simulink model "TestChaineAirNew"  (R2025a)
settings: Solver=ode45  StartTime=0.0  StopTime=SimuPumpStop  FixedStep=0.1  MaxStep=0.005  RelTol=1e-9  EnableMultiTasking=on
undefined symbols (not defined in the file): AirMotTest, AirPapTest, AirPressureTest, AirTimeTest, gam, Mim0, nv_remp, P0, Pamb, PcolPapTest, PRcrit, Rair, RegimeTest, SectionPapTest, Tamb, TempsPapTest, TempsTest, Vcyl
settings Model: Creator=a030141  LastModifiedBy=Hugo
settings SolverCC: AlgebraicLoopSolver=TrustRegion
settings DataIOCC: LimitDataPoints=on  SaveFormat=Array  SignalLoggingSaveFormat=ModelDataLogs  ReturnWorkspaceOutputs=off  SignalLoggingName=sigsOut
settings OptimizationCC: InitFltsAndDblsToZero=on  LifeSpan=inf
settings DebuggingCC: SaveWithParameterizedLinksMsg=none  UnderspecifiedInitializationDetection=Classic  MergeDetectMultiDrivingBlocksExec=none  SignalResolutionControl=TryResolveAllWithWarning  MultiTaskDSMMsg=warning  MultiTaskCondExecSysMsg=none  FcnCallInpInsideContextMsg=warning  UnconnectedInputMsg=warning  UnconnectedOutputMsg=warning  UnconnectedLineMsg=warning  SFUnexpectedBacktrackingDiag=warning  SFNoUnconditionalDefaultTransitionDiag=warning  SFExecutionAtInitializationDiag=none  ArithmeticOperatorsInVariantConditions=warning
settings HardwareCC: ProdBitPerPointer=32.0  ProdBitPerSizeT=32.0  ProdBitPerPtrDiffT=32.0  ProdLargestAtomicFloat=None  ProdIntDivRoundTo=Undefined  ProdEndianess=Unspecified  ProdWordSize=32.0  ProdHWDeviceType=32-bit Generic  TargetUnknown=on
settings ModelReferenceCC: PropagateSignalLabelsOutOfModel=off
settings RTWCC: GPUComputeCapability=3.5
settings CodeAppCC: StateflowObjectComments=on
settings GRTTargetCC: TargetFcnLib=ansi_tfl_tmw.mat  TargetLangStandard=C89/C90 (ANSI)  CombineOutputUpdateFcns=off  GRTInterface=on
settings ConfigComp: CovMetricSettings=dw  CovSaveCumulativeToWorkspaceVar=on  CovSaveSingleToWorkspaceVar=on

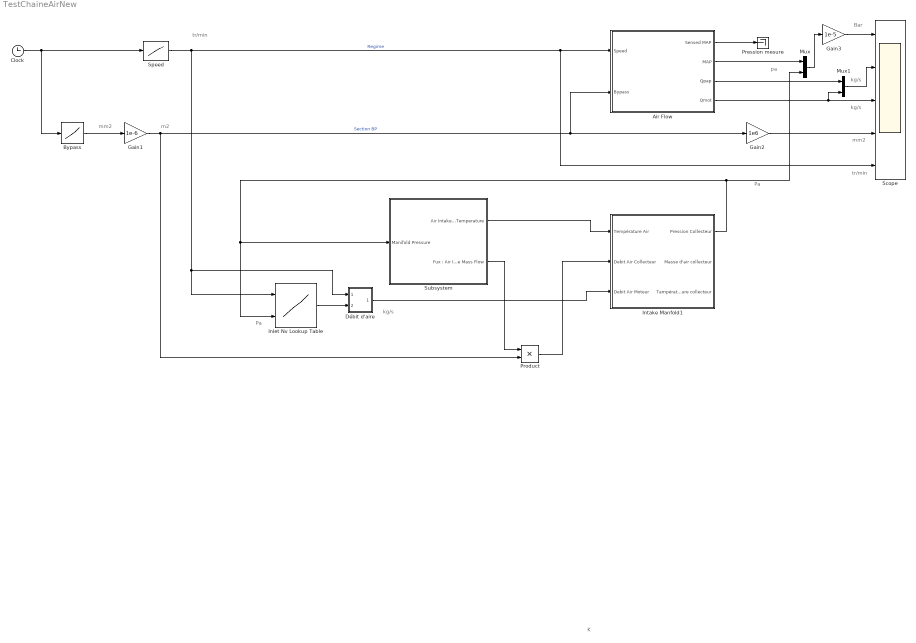
== system TestChaineAirNew ==
  note: pa
  note: Bar
  note: tr/min
  note: tr/min
  note: Pa
  note: m2
  note: mm2
  note: mm2
  note: kg/s
  note: kg/s
  note: Pa
  note: kg/s
  note: K
  Air Flow : Subsystem
  Bypass : Lookup  InputValues=TempsPapTest  Table=SectionPapTest.*PcolPapTest
  Clock : Clock
  Débit d'aire : Subsystem
  Gain1 : Gain  Gain=1e-6  SaturateOnIntegerOverflow=on  OutDataTypeStr=Inherit: Same as input  ParamDataTypeStr=Inherit: Same as input
  Gain2 : Gain  Gain=1e6  SaturateOnIntegerOverflow=on  OutDataTypeStr=Inherit: Same as input  ParamDataTypeStr=Inherit: Same as input
  Gain3 : Gain  Gain=1e-5  SaturateOnIntegerOverflow=on  OutDataTypeStr=Inherit: Same as input  ParamDataTypeStr=Inherit: Same as input
  Inlet Nv Lookup Table : Lookup2D  RowIndex=Ne_remp  ColumnIndex=Pcol_remp  Table=nv_remp
  Intake Manfold1 : Subsystem
  Mux : Mux  Inputs=2
  Mux1 : Mux  Inputs=2
  Pression mesure : Terminator
  Product : Product
  Scope : Scope  NumInputPorts=5
      settings: TimeSpan=374.5  Title=Pcol [bars]  ActiveDisplayYMinimum=0.769380841937612  ActiveDisplayYMaximum=1.0327907950597828
  Speed : Lookup  InputValues=TempsTest  Table=RegimeTest
  Subsystem : Subsystem
  wires:
  Clock/1 -> Speed/1, Bypass/1
  Bypass/1 -> Gain1/1
  Air Flow/2(MAP) -> Mux/1
  Mux/1 -> Gain3/1
  Gain3/1 -> Scope/1
  Air Flow/4(Qmot) -> Scope/3, Mux1/2
  Gain2/1 -> Scope/4
  Mux1/1 -> Scope/2
  Air Flow/1(Sensed MAP) -> Pression mesure/1
  Gain1/1 -> Gain2/1, Air Flow/2(Bypass), Product/2  "Section BP"
  Air Flow/3(Qpap) -> Mux1/1
  Speed/1 -> Scope/5, Air Flow/1(Speed), Débit d'aire/1(In1), Inlet Nv Lookup Table/1  "Regime"
  Débit d'aire/1(Debit Air Moteur) -> Intake Manfold1/3(Debit Air Moteur)
  Inlet Nv Lookup Table/1 -> Débit d'aire/2(In2)
  Subsystem/2("Fux : Air Intake Mass Flow") -> Product/1
  Product/1 -> Intake Manfold1/2(Debit Air Collecteur)
  Subsystem/1(Air Intake Temperature) -> Intake Manfold1/1(Température Air)
  Intake Manfold1/1(Pression Collecteur) -> Inlet Nv Lookup Table/2, Subsystem/1(Manifold Pressure), Mux/2

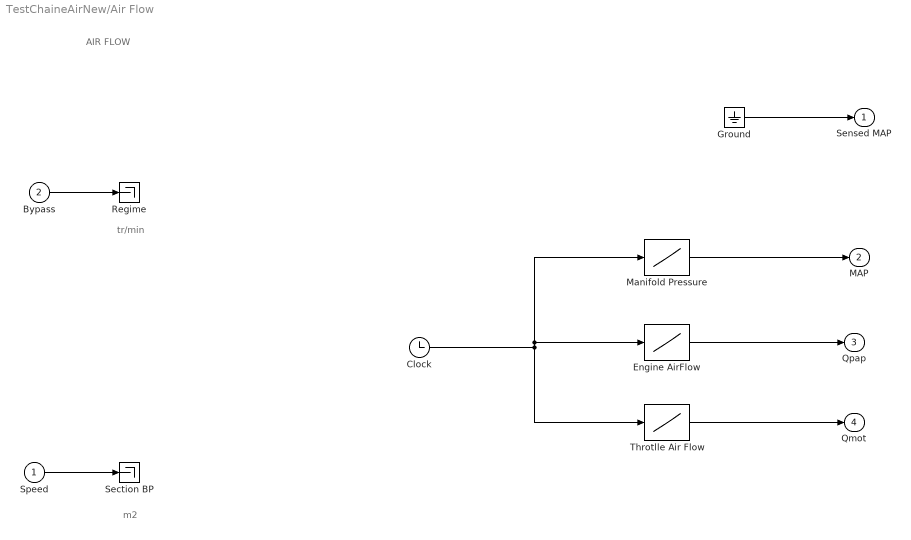
== system TestChaineAirNew/Air Flow ==
  note: AIR FLOW
  note: m2
  note: tr/min
  Speed : Inport
  Bypass : Inport  Port=2
  Clock : Clock
  Engine AirFlow : Lookup  InputValues=AirTimeTest  Table=AirMotTest
  Ground : Ground
  Manifold Pressure : Lookup  InputValues=AirTimeTest  Table=AirPressureTest
  Regime : Terminator
  Section BP : Terminator
  Throtlle Air Flow : Lookup  InputValues=AirTimeTest  Table=AirPapTest
  Sensed MAP : Outport
  MAP : Outport  Port=2
  Qpap : Outport  Port=3
  Qmot : Outport  Port=4
  wires:
  Bypass/1 -> Regime/1
  Speed/1 -> Section BP/1
  Ground/1 -> Sensed MAP/1
  Clock/1 -> Manifold Pressure/1, Engine AirFlow/1, Throtlle Air Flow/1
  Manifold Pressure/1 -> MAP/1
  Throtlle Air Flow/1 -> Qmot/1
  Engine AirFlow/1 -> Qpap/1

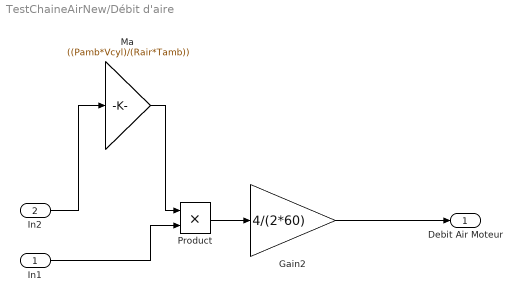
== system TestChaineAirNew/Débit d'aire ==
  In1 : Inport
  In2 : Inport  Port=2
  Gain2 : Gain  Gain=4/(2*60)
  Ma : Gain  Gain=((Pamb*Vcyl)/(Rair*Tamb))
  Product : Product
  Debit Air Moteur : Outport
  wires:
  Ma/1 -> Product/1
  Gain2/1 -> Debit Air Moteur/1
  Product/1 -> Gain2/1
  In1/1 -> Product/2
  In2/1 -> Ma/1

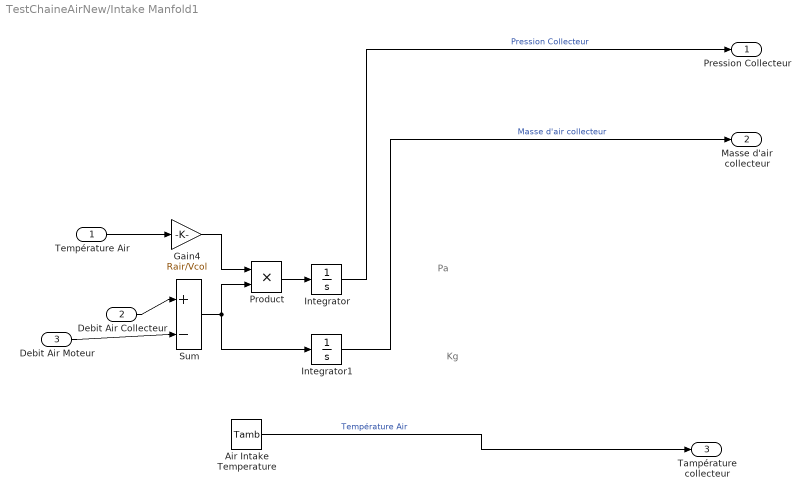
== system TestChaineAirNew/Intake Manfold1 ==
  note: Pa
  note: Kg
  Température Air : Inport
  Debit Air Collecteur : Inport  Port=2
  Debit Air Moteur : Inport  Port=3
  Air Intake Temperature : Constant  Value=Tamb
  Gain4 : Gain  Gain=Rair/Vcol
  Integrator : Integrator  InitialCondition=P0
  Integrator1 : Integrator  InitialCondition=Mim0
  Product : Product
  Sum : Sum  Inputs=|+-
  Pression Collecteur : Outport
  Masse d'air collecteur : Outport  Port=2
  Tampérature collecteur : Outport  Port=3
  wires:
  Gain4/1 -> Product/1
  Sum/1 -> Integrator1/1, Product/2
  Product/1 -> Integrator/1
  Température Air/1 -> Gain4/1
  Integrator1/1 -> Masse d'air collecteur/1  "Masse d'air collecteur"
  Debit Air Moteur/1 -> Sum/2
  Integrator/1 -> Pression Collecteur/1  "Pression Collecteur"
  Debit Air Collecteur/1 -> Sum/1
  Air Intake Temperature/1 -> Tampérature collecteur/1  "Température Air"

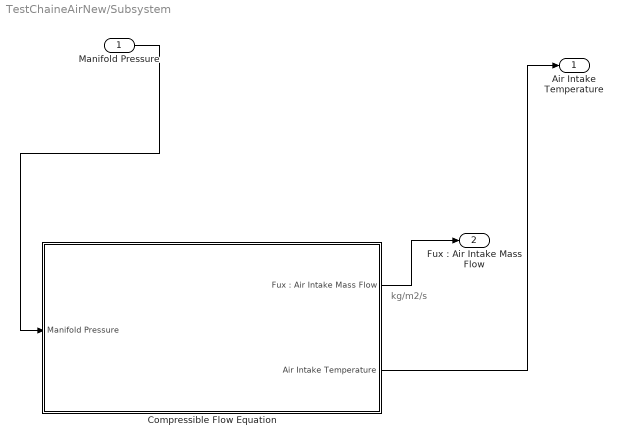
== system TestChaineAirNew/Subsystem ==
  note: kg/m2/s
  Manifold Pressure : Inport
  Compressible Flow Equation : Subsystem
  Air Intake Temperature : Outport
  "Fux : Air Intake Mass Flow" : Outport  Port=2
  wires:
  Compressible Flow Equation/2(Air Intake Temperature) -> Air Intake Temperature/1
  Manifold Pressure/1 -> Compressible Flow Equation/1(Manifold Pressure)
  Compressible Flow Equation/1("Fux : Air Intake Mass Flow") -> "Fux : Air Intake Mass Flow"/1

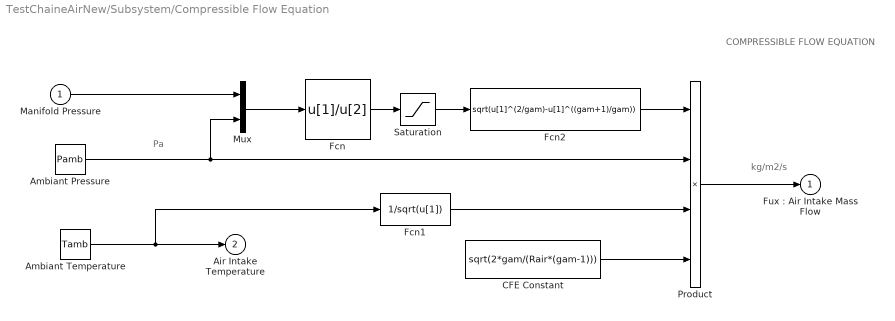
== system TestChaineAirNew/Subsystem/Compressible Flow Equation ==
  note: COMPRESSIBLE FLOW EQUATION
  note: Pa
  note: kg/m2/s
  Manifold Pressure : Inport
  Ambiant Pressure : Constant  Value=Pamb
  Ambiant Temperature : Constant  Value=Tamb
  "CFE Constant " : Constant  Value=sqrt(2*gam/(Rair*(gam-1)))
  Fcn : Fcn  Expr=u[1]/u[2]
  Fcn1 : Fcn  Expr=1/sqrt(u[1])
  Fcn2 : Fcn  Expr=sqrt(u[1]^(2/gam)-u[1]^((gam+1)/gam))
  Mux : Mux  Inputs=2
  Product : Product  Inputs=4  InputSameDT=on  SaturateOnIntegerOverflow=on  OutDataTypeStr=Inherit: Same as first input
  Saturation : Saturate  UpperLimit=1  LowerLimit=PRcrit
  "Fux : Air Intake Mass Flow" : Outport
  Air Intake Temperature : Outport  Port=2
  wires:
  Ambiant Pressure/1 -> Product/2, Mux/2
  Product/1 -> "Fux : Air Intake Mass Flow"/1
  "CFE Constant "/1 -> Product/4
  Fcn2/1 -> Product/1
  Saturation/1 -> Fcn2/1
  Fcn1/1 -> Product/3
  Fcn/1 -> Saturation/1
  Mux/1 -> Fcn/1
  Manifold Pressure/1 -> Mux/1
  Ambiant Temperature/1 -> Fcn1/1, Air Intake Temperature/1
